simulink model "untitled"  (R2020a)
settings: Solver=VariableStepAuto  StartTime=0.0  StopTime=10.0  RelTol=1e-3
settings Model: Creator=zoreacry  LastModifiedBy=zoreacry

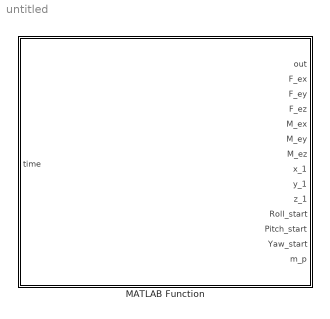
== system untitled ==
  MATLAB Function : MATLAB Function  TreatAsAtomicUnit=on

== matlab function untitled/MATLAB Function ==
  data: out output; F_ex output; F_ey output; F_ez output; M_ex output; M_ey output; M_ez output; x_1 output; y_1 output; z_1 output; Roll_start output; Pitch_start output; Yaw_start output; m_p output; time input
function [out,F_ex,F_ey,F_ez,M_ex,M_ey,M_ez,x_1,y_1,z_1,Roll_start,Pitch_start,Yaw_start,m_p]=position_get(time)

position=zeros(6,1000);
Velocity=zeros(6,1000);          %w位移速度与加速度位移数组
accelrate=zeros(6,1000);

%--------------------------------------------外力------------
F_ex=0;
F_ey=0;
F_ez=0;
M_ex=0;
M_ey=0;
M_ez=0;
p=1;
m_p=10;
%----------------------------------------初始位置的姿态------------------------------------

x_0 = 0;                                       %动平台 相对 静平台 的初始位置的坐标
y_0 = 0;                                       %可以改动，意为：更改初始时刻动平台相对于静平台的坐标
z_0 = 0;

%----------------------------------------动平台的位姿---------------------------

Roll = 0;                                      %相对静平台的姿态
Pitch = 0;                                     %可以改动，意为：更改初始时刻动平台相对于静平台的姿态
Yaw = 0;

%---------------------------------------其他设定------------------------------------

Roll_start = 10;                               %设定末端点的姿态
Pitch_start = 45;                              %可以改动，意为：更改为末端点的姿态
Yaw_start = 0;

x_1 = 450;                                       %设定末端点的位置
y_1 = 300;                                       %可以改动，意为：更改为末端点的位置
z_1 = 650;

target = sqrt((x_1 - x_0) ^ 2 + (y_1 - y_0) ^ 2 + (z_1 - z_0) ^ 2);           %计算所走位移
progress = 0;                                                                 %设定当前位移所走距离
currentvel = 0;                                                               %设定当前速度
time = 0;                                                                     %设定初始时刻

%=======================================以下都可以进行相应改动==========================%

cycle_time = 0.01;                                            %设定步长时间

maxaccel = 20;                                                 %设定最大加速度

feed_override = 1.2;                                          %设定倍率（进行瞬调）

maxvel = 10000;                                                %设定机床规定最大速度

reqvel = 150;                                                  %设定此用户给定的速度

hold on;

%----------------------------------------------------------------------------------------------

%---------------------------------平台基本尺寸（可以进行改动）---------------------------------

%--------------------------------------------------进行每次画图-------------------------------
while progress < target  %progress:当前位姿
    [progress, currentvel,newaccel] = tcRunCycle(progress, reqvel, currentvel,cycle_time,target,maxaccel, feed_override, maxvel);         %调用速度规划函数
    time = time + cycle_time;                                                       %进行时间迭代
    
    x_now = progress / target * (x_1 - x_0) + x_0;                                 %计算当前位置
    y_now = progress / target * (y_1 - y_0) + y_0;
    z_now = progress / target * (z_1 - z_0) + z_0;
    
    Roll_now_degree = (progress / target) * (Roll_start - Roll) + Roll;                    %计算当前角度
    Pitch_now_degree = (progress / target) * (Pitch_start - Pitch) + Pitch;
    Yaw_now_degree = (progress / target) * (Yaw_start - Yaw) + Yaw;
    
    P = [x_now;y_now;z_now];                                                       %动平台相对于静平台的实时位置
    
    TransM = [cosd(Pitch_now_degree) * cosd(Yaw_now_degree), sind(Roll_now_degree) * sind(Pitch_now_degree) * cosd(Yaw_now_degree) - cosd(Roll_now_degree) * sind(Yaw_now_degree), sind(Roll_now_degree) * sind(Yaw_now_degree) + cosd(Roll_now_degree) * sind(Pitch_now_degree) * cosd(Yaw_now_degree);cosd(Pitch_now_degree) * sind(Yaw_now_degree), cosd(Roll_now_degree) * cosd(Yaw_now_degree) + sind(Roll_now_degree) * sind(Pitch_now_degree) * sind(Yaw_now_degree), cosd(Roll_now_degree) * sind(Pitch_now_degree) * sind(Yaw_now_degree) - sind(Roll_now_degree) * cosd(Yaw_now_degree); - sind(Pitch_now_degree), sind(Roll_now_degree) * cosd(Pitch_now_degree), cosd(Roll_now_degree) * cosd(Pitch_now_degree)];
    %XYZ旋转矩阵
     
a_x=(newaccel/target)*(x_1-x_0);
a_y=(newaccel/target)*(y_1-y_0);
a_z=(newaccel/target)*(z_1-z_0);
omega_x_d=(newaccel/target)*(Roll_start-Roll);
omega_y_d=(newaccel/target)*(Pitch_start-Pitch);
omega_z_d=(newaccel/target)*(Yaw_start-Yaw);
v_x=(currentvel/target)*(x_1-x_0);
v_y=(currentvel/target)*(y_1-y_0);
v_z=(currentvel/target)*(z_1-z_0);
omega_x=(currentvel/target)*(Roll_start-Roll);
omega_y=(currentvel/target)*(Pitch_start-Pitch);
omega_z=(currentvel/target)*(Yaw_start-Yaw);

    position(1,p) =x_now;   position(2,p)=y_now;   position(3,p)=z_now;   position(4,p)=Roll_now_degree ;   position(5,p)=Pitch_now_degree ;   position(6,p)=Yaw_now_degree;%位置参数
    Velocity(1,p) =(currentvel/target)*(x_1-x_0);  Velocity(2,p) =(currentvel/target)*(y_1-y_0); Velocity(3,p) =(currentvel/target)*(z_1-z_0); Velocity(4,p) =(currentvel/target)*(Roll_start-Roll); Velocity(5,p) =(currentvel/target)*(Pitch_start-Pitch); Velocity(6,p) =(currentvel/target)*(Yaw_start-Yaw);         %w位移速度与加速度位移数组
    accelrate(1,p)=(newaccel/target)*(x_1-x_0); accelrate(2,p)=(newaccel/target)*(y_1-y_0); accelrate(3,p)=(newaccel/target)*(z_1-z_0); accelrate(4,p)=(newaccel/target)*(Roll_start-Roll); accelrate(5,p)=(newaccel/target)*(Pitch_start-Pitch); accelrate(6,p)=(newaccel/target)*(Yaw_start-Yaw);
    
  p=p+1;
  
end
u=7;
x_out=position(1,u);y_out=position(2,u);z_out=position(3,u);Roll_now_degree_out=position(4,u);Pitch_now_degree_out=position(5,u);Yaw_now_degree_out=position(6,u);
v_x_out=Velocity(1,u);v_y_out=Velocity(2,u);v_z_out=Velocity(3,u);v_roll_out=Velocity(4,u);v_pitch_out=Velocity(5,u);v_Yaw_out=Velocity(6,u);
a_x_out=accelrate(1,u);a_y_out=accelrate(2,u);a_z_out=accelrate(3,u);a_roll_out=accelrate(4,u);a_pitch_out=accelrate(5,u);a_Yaw_out=accelrate(6,u);

out=[x_out;y_out;z_out;Roll_now_degree_out;Pitch_now_degree_out;Yaw_now_degree_out;v_x_out;v_y_out;v_z_out;v_roll_out;v_pitch_out;v_Yaw_out;...
     a_x_out;a_y_out;a_z_out;a_roll_out;a_pitch_out;a_Yaw_out];
end
